simulink library "groundStationPrescribed001_cl"  (R2020a)
settings: Solver=VariableStepAuto  StartTime=0.0  StopTime=10.0  RelTol=1e-3
libraries: eulAng2RotMat_ul x1, thrAttachPtKinematics_ul x1
settings Model: Creator=M.Cobb  LastModifiedBy=andre
settings DataIOCC: ReturnWorkspaceOutputs=off
settings DebuggingCC: ArithmeticOperatorsInVariantConditions=warning
settings SFSimCC: CustomCodeUndefinedFunction=UseInterfaceOnly

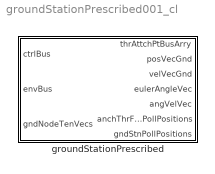
== system groundStationPrescribed001_cl ==
  groundStationPrescribed : Subsystem  mask{gs=0}
      mask prompts: gs "Ground station object"

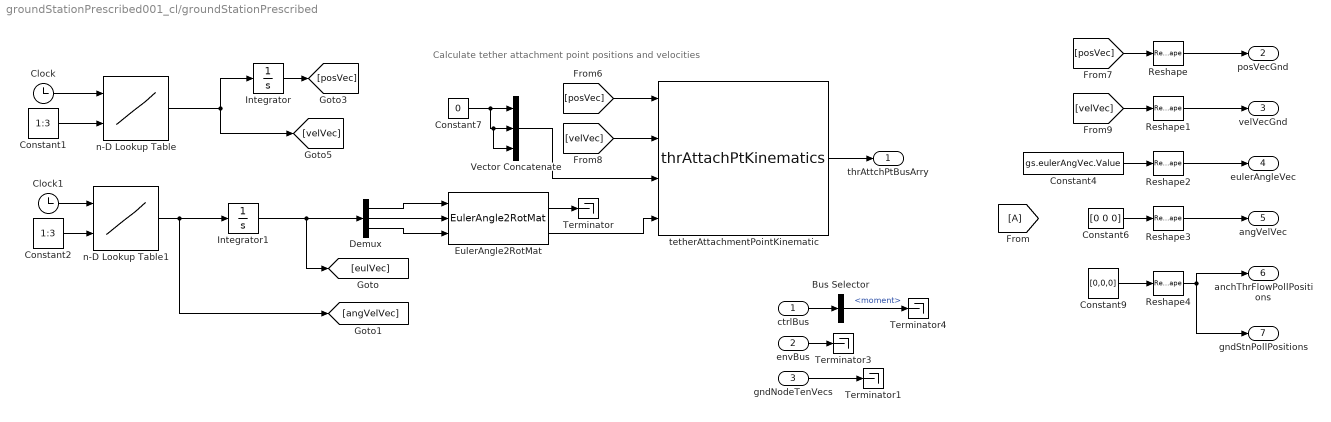
== system groundStationPrescribed001_cl/groundStationPrescribed ==
  note: Calculate tether attachment point positions and velocities
  ctrlBus : Inport  OutDataTypeStr=Bus: gndStnCtrlBus
  envBus : Inport  Port=2  OutDataTypeStr=Bus: envBus
  gndNodeTenVecs : Inport  Port=3
  Bus Selector : BusSelector  OutputSignals=moment
  Clock : Clock
  Clock1 : Clock
  Constant1 : Constant  Value=1:3
  Constant2 : Constant  Value=1:3
  Constant4 : Constant  Value=gs.eulerAngVec.Value
  Constant6 : Constant  Value=[0 0 0]
  Constant7 : Constant  Value=0
  Constant9 : Constant  Value=[0,0,0]
  Demux : Demux  Outputs=3
  EulerAngle2RotMat : eulAng2RotMat_ul/EulerAngle2RotMat  SystemSampleTime=-1  Latency=0  AutoFrameSizeCalculation=off
  Integrator : Integrator  InitialCondition=gs.initPosVec.Value
  Integrator1 : Integrator
  Reshape{,1..4} (5 alike) : Reshape  OutputDimensionality=Column vector (2-D)
  Terminator{,1,3..4} (4 alike) : Terminator
  Vector Concatenate : Concatenate  NumInputs=3
  n-D Lookup Table : Lookup_n-D  BreakpointsForDimension1=gs.velVecTrajectory.Value.Time  BreakpointsForDimension2=[1:3]  BreakpointsForDimension3=[5, 7]  Table=gs.velVecTrajectory.Value.Data  InternalRulePriority=Speed  RndMeth=Simplest  InputSameDT=on
  n-D Lookup Table1 : Lookup_n-D  BreakpointsForDimension1=gs.velVecTrajectory.Value.Time  BreakpointsForDimension2=[1:3]  BreakpointsForDimension3=[5, 7]  Table=gs.velVecTrajectory.Value.Data  InternalRulePriority=Speed  RndMeth=Simplest  InputSameDT=on
  tetherAttachmentPointKinematic : thrAttachPtKinematics_ul/thrAttachPtKinematics  atchPts=gs.struct('OCT.thrAttch')
  thrAttchPtBusArry : Outport  VectorParamsAs1DForOutWhenUnconnected=off
  posVecGnd : Outport  Port=2  VectorParamsAs1DForOutWhenUnconnected=off
  velVecGnd : Outport  Port=3  VectorParamsAs1DForOutWhenUnconnected=off
  eulerAngleVec : Outport  Port=4  VectorParamsAs1DForOutWhenUnconnected=off
  angVelVec : Outport  Port=5  VectorParamsAs1DForOutWhenUnconnected=off
  anchThrFlowPollPositions : Outport  Port=6  VectorParamsAs1DForOutWhenUnconnected=off
  gndStnPollPositions : Outport  Port=7  VectorParamsAs1DForOutWhenUnconnected=off
  wires:
  tetherAttachmentPointKinematic/1 -> thrAttchPtBusArry/1
  EulerAngle2RotMat/2 -> tetherAttachmentPointKinematic/4
  Vector Concatenate/1 -> tetherAttachmentPointKinematic/3
  Constant7/1 -> Vector Concatenate/1, Vector Concatenate/3, Vector Concatenate/2
  ctrlBus/1 -> Bus Selector/1
  envBus/1 -> Terminator3/1
  gndNodeTenVecs/1 -> Terminator1/1
  Reshape/1 -> posVecGnd/1
  Reshape1/1 -> velVecGnd/1
  Reshape2/1 -> eulerAngleVec/1
  Reshape3/1 -> angVelVec/1
  Constant6/1 -> Reshape3/1
  Bus Selector/1 -> Terminator4/1  "<moment>"
  Reshape4/1 -> anchThrFlowPollPositions/1, gndStnPollPositions/1
  Constant9/1 -> Reshape4/1
  Integrator/1 -> [posVec]
  [posVec] -> tetherAttachmentPointKinematic/1
  [posVec] -> Reshape/1
  [velVec] -> tetherAttachmentPointKinematic/2
  [velVec] -> Reshape1/1
  Clock/1 -> n-D Lookup Table/1
  n-D Lookup Table/1 -> [velVec], Integrator/1
  Constant1/1 -> n-D Lookup Table/2
  Constant4/1 -> Reshape2/1
  EulerAngle2RotMat/1 -> Terminator/1
  Integrator1/1 -> [eulVec], Demux/1
  Demux/3 -> EulerAngle2RotMat/3
  Demux/2 -> EulerAngle2RotMat/2
  Demux/1 -> EulerAngle2RotMat/1
  Clock1/1 -> n-D Lookup Table1/1
  Constant2/1 -> n-D Lookup Table1/2
  n-D Lookup Table1/1 -> [angVelVec], Integrator1/1
